simulink model "MSD_mask"  (R2022b)
settings: Solver=FixedStepAuto  StartTime=0.0  StopTime=60  FixedStep=0.001  RelTol=1e-6
PreLoadFcn:
  | % Initial Condition
  | m = 1;
  | b = 0.3;
  | k = 2;
  | 
  | % State-Space
  | A = [0 1; -k/m -b/m];
  | B = [0; 1/m];
  | C = [1 0];
  | D = 0;
  | 
  | % Transfer function
  | [Num, Den] = ss2tf(A,B,C,D);
settings Model: Creator=user  LastModifiedBy=user

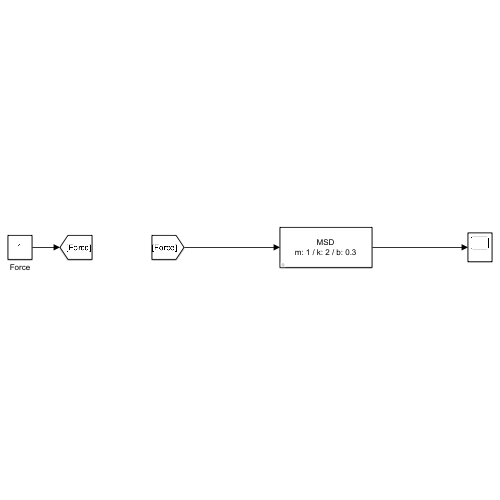
[thumbnail: Simulink's stored preview of the top-level diagram]
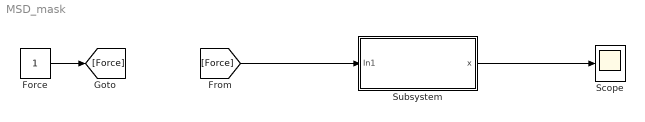
== system MSD_mask ==
  Force : Constant
  Scope : Scope
  Subsystem : Subsystem  mask{m=1, k=2, b=0.3}
      mask prompts: m "Mass [kg]"; k "Spring_Coefficient [k]"; b "Damping_Coefficient [b]"
      mask DialogControl ParameterGroupVar Prompt: 파라미터
      mask Display:
      | m = get_param(gcb,'m');
      | k = get_param(gcb,'k');
      | b = get_param(gcb,'b');
      | 
      | disp(['MSD\n' 'm: ' num2str(m) ' / k: ' num2str(k) ' / b: ' num2str(b)]);
  wires:
  Force/1 -> [Force]
  [Force] -> Subsystem/1(In1)
  Subsystem/1(x) -> Scope/1

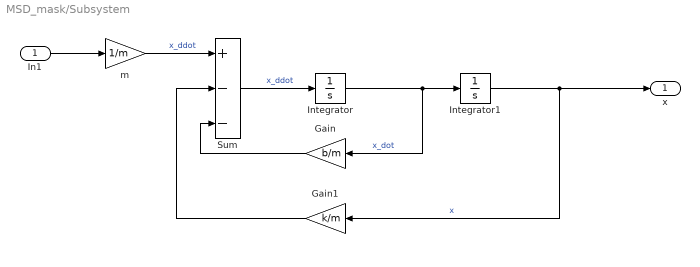
== system MSD_mask/Subsystem ==
  In1 : Inport
  Gain : Gain  Gain=b/m
  Gain1 : Gain  Gain=k/m
  Integrator : Integrator
  Integrator1 : Integrator
  Sum : Sum  Inputs=+--
  m : Gain  Gain=1/m
  x : Outport
  wires:
  Gain1/1 -> Sum/2
  Integrator/1 -> Gain/1, Integrator1/1  "x_dot"
  Sum/1 -> Integrator/1  "x_ddot"
  Gain/1 -> Sum/3
  Integrator1/1 -> x/1, Gain1/1  "x"
  In1/1 -> m/1
  m/1 -> Sum/1  "x_ddot"
